simulink model "First_HIL_Scenario2"  (R2023a)
settings: Solver=ode1  StartTime=0.0  StopTime=inf  FixedStep=0.001  RelTol=1e-3
undefined symbols (not defined in the file or in its folder): ACC_X, ACC_Y, ACC_Z, Altitude, distance, GetTimeDemo, Gyro_X, Gyro_Y, Gyro_Z, Heading, Lane_Car_Distance_Left, Lane_Car_Distance_Right, Lane_Class, Lane_Coefficient_C0, Lane_Coefficient_C1, Lane_Coefficient_C2, Lane_Coefficient_C3, Lane_Curvature, Lane_Distance, Lane_ID, Latitude, Longitude, OBJ_Class, OBJ_Height, OBJ_ID, OBJ_Length, OBJ_RCS, OBJ_S_Azimuth, OBJ_S_Elevation, OBJ_S_Range, OBJ_S_Velocity, OBJ_Velocity, OBJ_Width, OBJ_X, OBJ_Y, OBJ_Z, Pitch, Roll, Subsystem, time, Timestamp, TrafficLight_Direction, TrafficLight_State, TrafficLight_Timer, Velocity, width, x, x1, x2, x3, x4, y, y1, y2, y3, y4, Yaw
(part 4 of 4)

== system First_HIL_Scenario2/Veh_1/Algorithm/ControlSignalFilter/Subsystem3 ==
  global_valid : Inport
  global_value : Inport  Port=2
  valid : Inport  Port=3
  value : Inport  Port=4
  Add : Sum
  Constant : Constant  Value=0
  Switch : Switch  Threshold=1  SaturateOnIntegerOverflow=off  InputSameDT=off
  Switch1 : Switch  Criteria=u2 > Threshold  SaturateOnIntegerOverflow=off  InputSameDT=off
  Switch2 : Switch  Criteria=u2 > Threshold  SaturateOnIntegerOverflow=off  InputSameDT=off
  disable : Constant  Value=0
  enable : Constant
  enable_out : Outport
  value_out : Outport  Port=2
  wires:
  global_valid/1 -> Switch1/2, Add/1
  valid/1 -> Switch2/2, Add/2
  Add/1 -> Switch/2
  enable/1 -> Switch/1
  disable/1 -> Switch/3
  Switch/1 -> enable_out/1
  global_value/1 -> Switch1/1
  value/1 -> Switch2/1
  Constant/1 -> Switch1/3
  Switch1/1 -> Switch2/3
  Switch2/1 -> value_out/1

== system First_HIL_Scenario2/Veh_1/Algorithm/ControlSignalFilter/Subsystem4 ==
  global_valid : Inport
  global_value : Inport  Port=2
  valid : Inport  Port=3
  value : Inport  Port=4
  Add : Sum
  Constant : Constant  Value=0
  Switch : Switch  Threshold=1  SaturateOnIntegerOverflow=off  InputSameDT=off
  Switch1 : Switch  Criteria=u2 > Threshold  SaturateOnIntegerOverflow=off  InputSameDT=off
  Switch2 : Switch  Criteria=u2 > Threshold  SaturateOnIntegerOverflow=off  InputSameDT=off
  disable : Constant  Value=0
  enable : Constant
  enable_out : Outport
  value_out : Outport  Port=2
  wires:
  global_valid/1 -> Switch1/2, Add/1
  valid/1 -> Switch2/2, Add/2
  Add/1 -> Switch/2
  enable/1 -> Switch/1
  disable/1 -> Switch/3
  Switch/1 -> enable_out/1
  global_value/1 -> Switch1/1
  value/1 -> Switch2/1
  Constant/1 -> Switch1/3
  Switch1/1 -> Switch2/3
  Switch2/1 -> value_out/1

== system First_HIL_Scenario2/Veh_1/VehicleDataBus/GlobalVariableWrite/GlobalVariableSwitch0 ==
  value : Inport
  time : Inport  Port=2
  originalValue : Inport  Port=3
  originalTIme : Inport  Port=4
  GlobalVariable0 : S-Function  FunctionName=DataSender  Parameters='global.0','time@i,variable@d','0.01','0.0','192.168.2.101','25010'  SFunctionDeploymentMode=off  EnableBusSupport=off
  Minus : Sum  Inputs=+-
  Switch : Switch  Criteria=u2 ~= 0  SaturateOnIntegerOverflow=off  InputSameDT=off
  wires:
  Switch/1 -> GlobalVariable0/1
  Minus/1 -> Switch/2
  time/1 -> Switch/1
  originalTIme/1 -> Switch/3
  originalValue/1 -> Minus/2
  value/1 -> Minus/1, GlobalVariable0/2

== system First_HIL_Scenario2/Veh_1/VehicleDataBus/GlobalVariableWrite/GlobalVariableSwitch1 ==
  value : Inport
  time : Inport  Port=2
  originalValue : Inport  Port=3
  originalTIme : Inport  Port=4
  GlobalVariable1 : S-Function  FunctionName=DataSender  Parameters='global.1','time@i,variable@d','0.01','0.0','192.168.2.101','25011'  SFunctionDeploymentMode=off  EnableBusSupport=off
  Minus : Sum  Inputs=+-
  Switch : Switch  Criteria=u2 ~= 0  SaturateOnIntegerOverflow=off  InputSameDT=off
  wires:
  Switch/1 -> GlobalVariable1/1
  Minus/1 -> Switch/2
  time/1 -> Switch/1
  originalTIme/1 -> Switch/3
  originalValue/1 -> Minus/2
  value/1 -> Minus/1, GlobalVariable1/2

== system First_HIL_Scenario2/Veh_1/VehicleDataBus/GlobalVariableWrite/GlobalVariableSwitch2 ==
  value : Inport
  time : Inport  Port=2
  originalValue : Inport  Port=3
  originalTIme : Inport  Port=4
  GlobalVariable2 : S-Function  FunctionName=DataSender  Parameters='global.2','time@i,variable@d','0.01','0.0','192.168.2.101','25012'  SFunctionDeploymentMode=off  EnableBusSupport=off
  Minus : Sum  Inputs=+-
  Switch : Switch  Criteria=u2 ~= 0  SaturateOnIntegerOverflow=off  InputSameDT=off
  wires:
  Switch/1 -> GlobalVariable2/1
  Minus/1 -> Switch/2
  time/1 -> Switch/1
  originalTIme/1 -> Switch/3
  originalValue/1 -> Minus/2
  value/1 -> Minus/1, GlobalVariable2/2

== system First_HIL_Scenario2/Veh_1/VehicleDataBus/GlobalVariableWrite/GlobalVariableSwitch3 ==
  value : Inport
  time : Inport  Port=2
  originalValue : Inport  Port=3
  originalTIme : Inport  Port=4
  GlobalVariable3 : S-Function  FunctionName=DataSender  Parameters='global.3','time@i,variable@d','0.01','0.0','192.168.2.101','25013'  SFunctionDeploymentMode=off  EnableBusSupport=off
  Minus : Sum  Inputs=+-
  Switch : Switch  Criteria=u2 ~= 0  SaturateOnIntegerOverflow=off  InputSameDT=off
  wires:
  Switch/1 -> GlobalVariable3/1
  Minus/1 -> Switch/2
  time/1 -> Switch/1
  originalTIme/1 -> Switch/3
  originalValue/1 -> Minus/2
  value/1 -> Minus/1, GlobalVariable3/2

== system First_HIL_Scenario2/Veh_1/VehicleDataBus/GlobalVariableWrite/GlobalVariableSwitch4 ==
  value : Inport
  time : Inport  Port=2
  originalValue : Inport  Port=3
  originalTIme : Inport  Port=4
  GlobalVariable4 : S-Function  FunctionName=DataSender  Parameters='global.4','time@i,variable@d','0.01','0.0','192.168.2.101','25014'  SFunctionDeploymentMode=off  EnableBusSupport=off
  Minus : Sum  Inputs=+-
  Switch : Switch  Criteria=u2 ~= 0  SaturateOnIntegerOverflow=off  InputSameDT=off
  wires:
  Switch/1 -> GlobalVariable4/1
  Minus/1 -> Switch/2
  time/1 -> Switch/1
  originalTIme/1 -> Switch/3
  originalValue/1 -> Minus/2
  value/1 -> Minus/1, GlobalVariable4/2

== system First_HIL_Scenario2/Veh_1/VehicleDataBus/GlobalVariableWrite/GlobalVariableSwitch5 ==
  value : Inport
  time : Inport  Port=2
  originalValue : Inport  Port=3
  originalTIme : Inport  Port=4
  GlobalVariable5 : S-Function  FunctionName=DataSender  Parameters='global.5','time@i,variable@d','0.01','0.0','192.168.2.101','25015'  SFunctionDeploymentMode=off  EnableBusSupport=off
  Minus : Sum  Inputs=+-
  Switch : Switch  Criteria=u2 ~= 0  SaturateOnIntegerOverflow=off  InputSameDT=off
  wires:
  Switch/1 -> GlobalVariable5/1
  Minus/1 -> Switch/2
  time/1 -> Switch/1
  originalTIme/1 -> Switch/3
  originalValue/1 -> Minus/2
  value/1 -> Minus/1, GlobalVariable5/2

== system First_HIL_Scenario2/Veh_1/VehicleDataBus/GlobalVariableWrite/GlobalVariableSwitch6 ==
  value : Inport
  time : Inport  Port=2
  originalValue : Inport  Port=3
  originalTIme : Inport  Port=4
  GlobalVariable6 : S-Function  FunctionName=DataSender  Parameters='global.6','time@i,variable@d','0.01','0.0','192.168.2.101','25016'  SFunctionDeploymentMode=off  EnableBusSupport=off
  Minus : Sum  Inputs=+-
  Switch : Switch  Criteria=u2 ~= 0  SaturateOnIntegerOverflow=off  InputSameDT=off
  wires:
  Switch/1 -> GlobalVariable6/1
  Minus/1 -> Switch/2
  time/1 -> Switch/1
  originalTIme/1 -> Switch/3
  originalValue/1 -> Minus/2
  value/1 -> Minus/1, GlobalVariable6/2

== system First_HIL_Scenario2/Veh_1/VehicleDataBus/GlobalVariableWrite/GlobalVariableSwitch7 ==
  value : Inport
  time : Inport  Port=2
  originalValue : Inport  Port=3
  originalTIme : Inport  Port=4
  GlobalVariable7 : S-Function  FunctionName=DataSender  Parameters='global.7','time@i,variable@d','0.01','0.0','192.168.2.101','25017'  SFunctionDeploymentMode=off  EnableBusSupport=off
  Minus : Sum  Inputs=+-
  Switch : Switch  Criteria=u2 ~= 0  SaturateOnIntegerOverflow=off  InputSameDT=off
  wires:
  Switch/1 -> GlobalVariable7/1
  Minus/1 -> Switch/2
  time/1 -> Switch/1
  originalTIme/1 -> Switch/3
  originalValue/1 -> Minus/2
  value/1 -> Minus/1, GlobalVariable7/2

== system First_HIL_Scenario2/Veh_1/VehicleDataBus/GlobalVariableWrite/GlobalVariableSwitch8 ==
  value : Inport
  time : Inport  Port=2
  originalValue : Inport  Port=3
  originalTIme : Inport  Port=4
  GlobalVariable8 : S-Function  FunctionName=DataSender  Parameters='global.8','time@i,variable@d','0.01','0.0','192.168.2.101','25018'  SFunctionDeploymentMode=off  EnableBusSupport=off
  Minus : Sum  Inputs=+-
  Switch : Switch  Criteria=u2 ~= 0  SaturateOnIntegerOverflow=off  InputSameDT=off
  wires:
  Switch/1 -> GlobalVariable8/1
  Minus/1 -> Switch/2
  time/1 -> Switch/1
  originalTIme/1 -> Switch/3
  originalValue/1 -> Minus/2
  value/1 -> Minus/1, GlobalVariable8/2

== system First_HIL_Scenario2/Veh_1/VehicleDataBus/GlobalVariableWrite/GlobalVariableSwitch9 ==
  value : Inport
  time : Inport  Port=2
  originalValue : Inport  Port=3
  originalTIme : Inport  Port=4
  GlobalVariable9 : S-Function  FunctionName=DataSender  Parameters='global.9','time@i,variable@d','0.01','0.0','192.168.2.101','25019'  SFunctionDeploymentMode=off  EnableBusSupport=off
  Minus : Sum  Inputs=+-
  Switch : Switch  Criteria=u2 ~= 0  SaturateOnIntegerOverflow=off  InputSameDT=off
  wires:
  Switch/1 -> GlobalVariable9/1
  Minus/1 -> Switch/2
  time/1 -> Switch/1
  originalTIme/1 -> Switch/3
  originalValue/1 -> Minus/2
  value/1 -> Minus/1, GlobalVariable9/2
